simulink model "sl_drivepose_vs"  (Simulink 8.4)
settings: Solver=ode45  StartTime=0.0  StopTime=10  MaxStep=0.05  RelTol=1e-3
InitFcn:
  | camera = CentralCamera('default', 'focal', 0.002);
  | P = [4 10 3; 9 9 2; 6 8 3; 8 10 4; 10 7 2]';
  | T_VC = transl(0.2, 0.1, 0.5)*troty(pi/2)*trotz(-pi/2);
  | x0 = [2 2 0];
  | xg = [5 5 pi/2];
undefined symbols (not defined in the file or in its folder): se2, se3
libraries: roblocks x6, simulink x1
settings Model: Creator=pic  LastModifiedBy=corkep
settings DataIOCC: LimitDataPoints=off  SaveState=on  ReturnWorkspaceOutputs=on

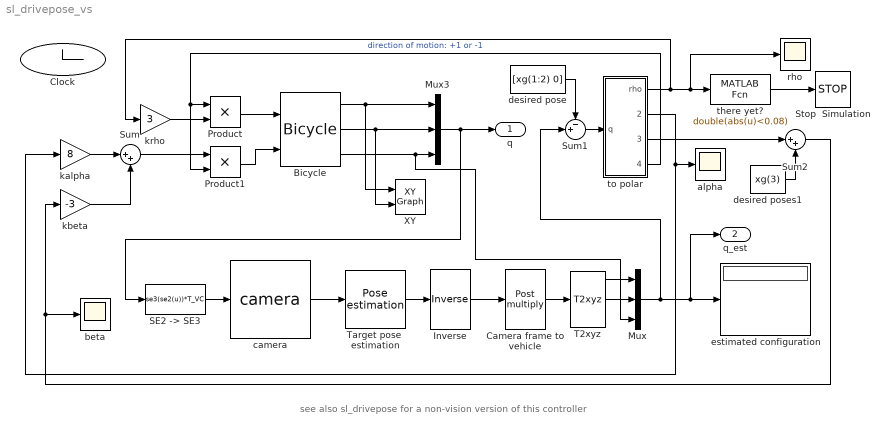
== system sl_drivepose_vs ==
  note: see also sl_drivepose for a non-vision version of this controller
  Bicycle : roblocks/Dynamics/Bicycle  accel=1  vlim=1  alim=1  L=1  x0=x0  handbrake=0
  Camera frame to vehicle : roblocks/Transform/Post multiply  T2=inv(T_VC)
  Clock : Clock
  Inverse : roblocks/Transform/Inverse
  Mux : Mux  Inputs=3
  Mux3 : Mux  Inputs=3
  Product : Product  RndMeth=Zero
  Product1 : Product  RndMeth=Zero
  "SE2 -> SE3" : MATLABFcn  MATLABFcn=se3(se2(u))*T_VC  Output1D=off
  Stop  Simulation : Stop
  Sum : Sum  Inputs=|++
  Sum1 : Sum  Inputs=-+|
  Sum2 : Sum  Inputs=|++
  T2xyz : roblocks/Transform Conversion/T2xyz
  Target pose  estimation : roblocks/Vision/Pose estimation  cam=camera  P=P
  XY : simulink/Sinks/XY Graph  xmin=-10  xmax=10  ymin=-10  ymax=10  st=-1
  alpha : Scope
      settings: TimeRange=4  YMin=-2  YMax=1
  beta : Scope
      settings: TimeRange=4  YMin=-1  YMax=2.5
  camera : roblocks/Vision/camera  cam=camera  points=P
  desired pose : Constant  Value=[xg(1:2) 0]
  desired poses1 : Constant  Value=xg(3)
  estimated configuration : Display
  kalpha : Gain  Gain=8
  kbeta : Gain  Gain=-3
  krho : Gain  Gain=3
  rho : Scope
      settings: TimeRange=4  YMin=1  YMax=3.25  SaveName=ScopeData2
  there yet? : MATLABFcn  MATLABFcn=double(abs(u)<0.08)  OutputSignalType=real
  to polar : Subsystem
  q : Outport
  q_est : Outport  Port=2
  wires:
  Mux3/1 -> q/1, "SE2 -> SE3"/1
  Bicycle/1 -> Mux3/1, XY/1
  Bicycle/2 -> Mux3/2, XY/2
  Bicycle/3 -> Mux3/3, Mux/3
  to polar/2(alpha) -> kalpha/1, alpha/1
  kalpha/1 -> Sum/1
  kbeta/1 -> Sum/2
  krho/1 -> Product/2
  to polar/1(rho) -> krho/1, there yet?/1, rho/1
  desired pose/1 -> Sum1/1
  Sum1/1 -> to polar/1(q)
  Sum/1 -> Product1/1
  there yet?/1 -> Stop  Simulation/1
  to polar/3(beta) -> Sum2/1
  Sum2/1 -> kbeta/1, beta/1
  desired poses1/1 -> Sum2/2
  "SE2 -> SE3"/1 -> camera/1
  camera/1 -> Target pose  estimation/1
  Target pose  estimation/1 -> Inverse/1
  Camera frame to vehicle/1 -> T2xyz/1
  T2xyz/1 -> Mux/1
  T2xyz/2 -> Mux/2
  Mux/1 -> estimated configuration/1, q_est/1, Sum1/2
  to polar/4(direction) -> Product1/2, Product/1  "direction of motion: +1 or -1"
  Inverse/1 -> Camera frame to vehicle/1
  Product/1 -> Bicycle/1
  Product1/1 -> Bicycle/2

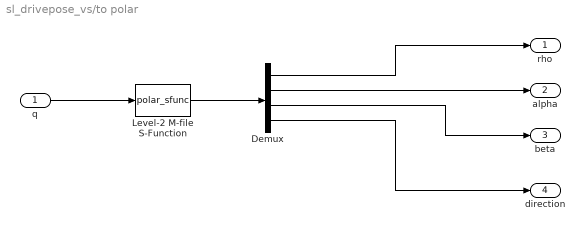
== system sl_drivepose_vs/to polar ==
  q : Inport
  Demux : Demux
  Level-2 M-file S-Function : M-S-Function  FunctionName=polar_sfunc
  rho : Outport
  alpha : Outport  Port=2
  beta : Outport  Port=3
  direction : Outport  Port=4
  wires:
  Demux/3 -> beta/1
  q/1 -> Level-2 M-file S-Function/1
  Level-2 M-file S-Function/1 -> Demux/1
  Demux/1 -> rho/1
  Demux/2 -> alpha/1
  Demux/4 -> direction/1
